simulink model "beluga_control_a"  (R2016a)
settings: Solver=FixedStepAuto  SolverMode=SingleTasking  StartTime=0.0  StopTime=10.0  FixedStep=0.001  RelTol=1e-3
values from neighbouring files (symbols this model uses):
  Ix = 0.05    [belugaSimulation.m]    (also in belugaStep.m; iverSimulation.m = 0; matlab.mat)
  Iy = 2.05    [belugaSimulation.m]    (also in belugaStep.m; iverSimulation.m = 0; matlab.mat)
  Iz = 2.06    [belugaSimulation.m]    (also in belugaStep.m; iverSimulation.m = 0; matlab.mat)
  K_pdot = -0.0704    [belugaSimulation.m]    (also in belugaStep.m; iverSimulation.m = 0; matlab.mat)
  m = 16.7/2.2    (= 7.59090909091)    [belugaSimulation.m]    (also in belugaStep.m = 4.2173; gps_state_est.m = 1; iverSimulation.m = 0; lin_test.m = 20.2)
  M_qdot = -3.2455    [belugaSimulation.m]    (also in belugaStep.m; iverSimulation.m = 0; matlab.mat)
  M_wdot = 2.5656    [belugaSimulation.m]    (also in belugaStep.m; iverSimulation.m = 0; matlab.mat)
  N_rdot = -3.2455    [belugaSimulation.m]    (also in belugaStep.m; iverSimulation.m = 0; matlab.mat)
  N_vdot = -2.5656    [belugaSimulation.m]    (also in belugaStep.m; iverSimulation.m = 0; matlab.mat)
  X_udot = -0.51334    [belugaSimulation.m]    (also in belugaStep.m; iverSimulation.m = 0; matlab.mat)
  xg = 0    [belugaSimulation.m]    (also in belugaStep.m; iverSimulation.m; matlab.mat)
  Y_rdot = -2.5656    [belugaSimulation.m]    (also in belugaStep.m; iverSimulation.m = 0; matlab.mat)
  Y_vdot = -23.8314    [belugaSimulation.m]    (also in belugaStep.m; iverSimulation.m = 0; matlab.mat)
  Z_qdot = 2.5656    [belugaSimulation.m]    (also in belugaStep.m; iverSimulation.m = 0; matlab.mat)
  Z_wdot = -23.8314    [belugaSimulation.m]    (also in belugaStep.m; iverSimulation.m = 0; matlab.mat)
  zg = 0    [belugaSimulation.m]    (also in belugaStep.m; iverSimulation.m; matlab.mat)
libraries: dspinverses x1
settings Model: Creator=HMCLoaner  LastModifiedBy=chriskotcherha
settings DebuggingCC: SFUnexpectedBacktrackingDiag=error  SFNoUnconditionalDefaultTransitionDiag=error
settings GRTTargetCC: TargetLangStandard=C99 (ISO)  GeneratePreprocessorConditionals=Use local settings
settings ConfigComp: CovMetricSettings=dwe  CovHtmlReporting=off  CovSaveCumulativeToWorkspaceVar=off  CovSaveSingleToWorkspaceVar=off  CovExternalEMLEnable=on

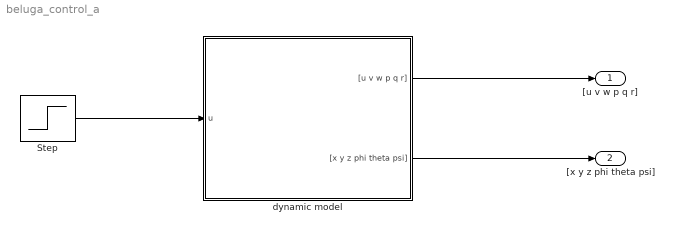
== system beluga_control_a ==
  Step : Step  Time=0  Before=[0 0 0 0]  After=1*[1 1 1 1]  SampleTime=0
  "dynamic model " : Subsystem
  "[u v w p q r]" : Outport
  "[x y z phi theta psi]" : Outport  Port=2
  wires:
  Step/1 -> "dynamic model "/1(u)
  "dynamic model "/1("[u v w p q r]") -> "[u v w p q r]"/1
  "dynamic model "/2("[x y z phi theta psi]") -> "[x y z phi theta psi]"/1

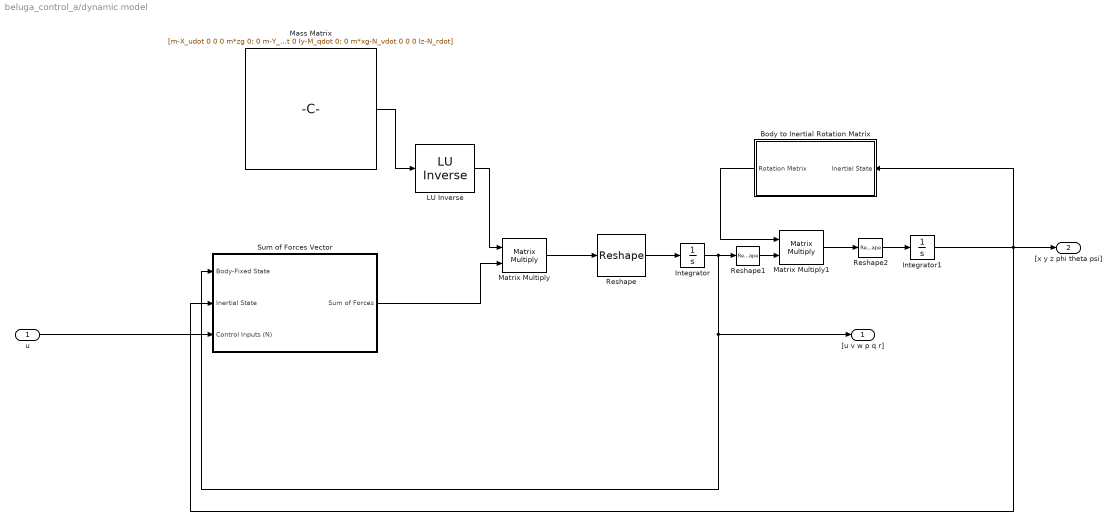
== system beluga_control_a/dynamic model  ==
  u : Inport  PortDimensions=[4,1]
  " LU Inverse" : dspinverses/ LU Inverse
  Body to Inertial Rotation Matrix : Subsystem
  Integrator : Integrator  InitialCondition=[0 0 0 0 0 0]'
  Integrator1 : Integrator  InitialCondition=[0 0 0 0 0 0]'
  "Mass Matrix " : Constant  Value=[m-X_udot 0 0 0 m*zg 0; 0 m-Y_vdot 0 -m*zg 0 m*xg-Y_rdot; 0 0 m-Z_wdot 0 -m*xg-Z_qdot 0; 0 -m*zg 0 Ix-K_pdot 0 0; m*zg 0 -m*xg-M_wdot 0 Iy-M_qdot 0; 0 m*xg-N_vdot 0 0 0 Iz-N_rdot]  VectorParams1D=off
  Matrix Multiply : Product  Multiplication=Matrix(*)
  Matrix Multiply1 : Product  Multiplication=Matrix(*)
  Reshape : Reshape  OutputDimensions=3
  Reshape1 : Reshape  OutputDimensions=[1,6]
  Reshape2 : Reshape  OutputDimensions=[6,1]
  Sum of Forces Vector : Subsystem
  "[u v w p q r]" : Outport
  "[x y z phi theta psi]" : Outport  Port=2
  wires:
  Matrix Multiply/1 -> Reshape/1
  Integrator/1 -> "[u v w p q r]"/1, Sum of Forces Vector/1(Body-Fixed State), Reshape1/1
  " LU Inverse"/1 -> Matrix Multiply/1
  Reshape1/1 -> Matrix Multiply1/2
  Matrix Multiply1/1 -> Reshape2/1
  Reshape2/1 -> Integrator1/1
  "Mass Matrix "/1 -> " LU Inverse"/1
  Body to Inertial Rotation Matrix/1(Rotation Matrix) -> Matrix Multiply1/1
  Sum of Forces Vector/1(Sum of Forces) -> Matrix Multiply/2
  u/1 -> Sum of Forces Vector/3(Control Inputs (N))
  Integrator1/1 -> "[x y z phi theta psi]"/1, Sum of Forces Vector/2(Inertial State), Body to Inertial Rotation Matrix/1(Inertial State)
  Reshape/1 -> Integrator/1

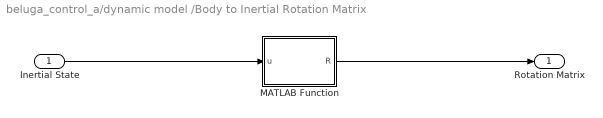
== system beluga_control_a/dynamic model /Body to Inertial Rotation Matrix ==
  Inertial State : Inport
  MATLAB Function : MATLAB Function  TreatAsAtomicUnit=on
  Rotation Matrix : Outport  PortDimensions=[6,6]
  wires:
  MATLAB Function/1(R) -> Rotation Matrix/1
  Inertial State/1 -> MATLAB Function/1(u)

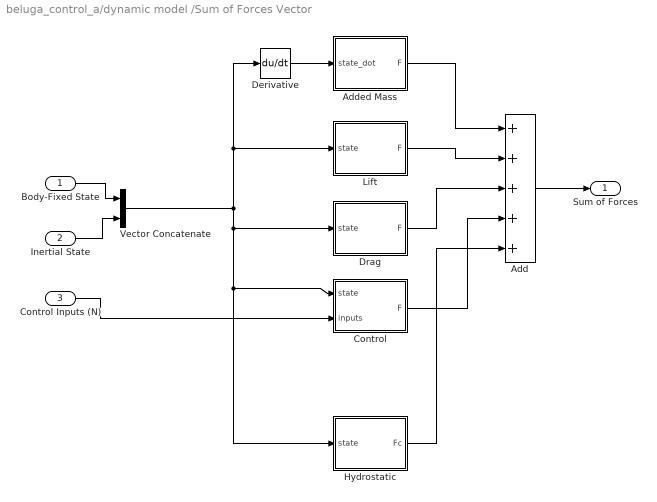
== system beluga_control_a/dynamic model /Sum of Forces Vector ==
  Body-Fixed State : Inport
  Inertial State : Inport  Port=2
  Control Inputs (N) : Inport  Port=3
  Add : Sum  Inputs=+++++
  Added Mass : MATLAB Function  TreatAsAtomicUnit=on
  Control : MATLAB Function  TreatAsAtomicUnit=on
  Derivative : Derivative
  Drag : MATLAB Function  TreatAsAtomicUnit=on
  Hydrostatic : MATLAB Function  TreatAsAtomicUnit=on
  Lift : MATLAB Function  TreatAsAtomicUnit=on
  Vector Concatenate : Concatenate
  Sum of Forces : Outport
  wires:
  Body-Fixed State/1 -> Vector Concatenate/1
  Inertial State/1 -> Vector Concatenate/2
  Vector Concatenate/1 -> Drag/1(state), Control/1(state), Hydrostatic/1(state), Derivative/1, Lift/1(state)
  Control Inputs (N)/1 -> Control/2(inputs)
  Hydrostatic/1(Fc) -> Add/5
  Add/1 -> Sum of Forces/1
  Control/1(F) -> Add/4
  Drag/1(F) -> Add/3
  Lift/1(F) -> Add/2
  Added Mass/1(F) -> Add/1
  Derivative/1 -> Added Mass/1(state_dot)

== matlab function beluga_control_a/dynamic model /Sum of Forces Vector/Control ==
  data: state input; F output; inputs input
function F = fcn(state, inputs)
    
    %% Constants TODO
        % TODO #1: Add in multiplying the sum of forces by r when
        %           calculating K_c
        % TODO #2: Check constants and polarity for K_c
        % TODO #3: Check M_c
        % TODO #4: Check polarity of N_c
        % TODO #5: Add in multiplying the sum of forces by L when
        %           calculating M_c
        % TODO #6: Add in multiplying the sum of forces by L when
        %           calculating N_c    
    %% Thruster Model
    % Values from documentation stationary calibration
    thruster_pwm = [1100        1110        1120        1130        1140        1150        1160        1170 1180        1190        1200        1210        1220        1230        1240        1250        1260        1270        1280        1290        1300        1310        1320        1330        1340        1350        1360        1370        1380        1390        1400        1410         1420        1430        1440        1450        1460        1470        1480        1490 1500        1510        1520        1530        1540        1550        1560        1570 1580        1590        1600        1610        1620        1630        1640        1650 1660        1670        1680        1690        1700        1710        1720        1730 1740        1750        1760        1770        1780        1790        1800        1810 1820        1830        1840        1850        1860        1870        1880        1890 1900];
    thruster_force = 9.81*[-4.0823   -4.0823   -4.0869   -3.8283   -3.7331   -3.6197   -3.4428   -3.3022   -3.1842   -3.0572 -2.9075   -2.8168   -2.7079   -2.5265   -2.3632   -2.2589   -2.1772   -1.9913   -1.8824   -1.7690 -1.6420   -1.4923   -1.3336   -1.2428   -1.1204   -1.0251   -0.9072   -0.7893   -0.6940   -0.6169 -0.5216   -0.4354   -0.3538   -0.2767   -0.1905   -0.1134   -0.0544   -0.0272         0         0 0         0         0    0.0590    0.1134    0.1860    0.2631    0.3493    0.4173    0.5216 0.6350    0.7167    0.8437    0.9435    1.1022    1.2474    1.3925    1.5286    1.6783    1.8053 1.9595    2.0956    2.2181    2.4131    2.5220    2.6943    2.8259    3.0209    3.1933    3.3521 3.4473    3.4927    3.7784    3.9417    4.0052    4.1957    4.3772    4.5677    4.8035    4.8988 5.0938];
    
    
    % From Arduino implementation
    DEAD_POS = 16;
    DEAD_NEG = -35;
    PERIOD = 500; % [ms]
    LEAK_THRESH = 150;
    
    %Correct for deadzone
    for i = 1:numel(inputs)
        if inputs(i) > 0
            inputs(i) = inputs(i)*50+DEAD_POS;
        elseif inputs(i) < 0
            inputs(i) = inputs(i)*50+DEAD_NEG;            
        end
        
        inputs(i) = inputs(i) + 1500;
        inputs(i) = interp1(thruster_pwm, thruster_force, inputs(i)); % assuming static thrust
    end


    %% States and calculations
    % defining states
    u = state(1); % x - velocity
    v = state(2); % y - velocity
    w = state(3); % z - velocity
    p = state(4); % angular velocity around the x-axis (velocity of phi)
    q = state(5); % angular velocity around the y-axis (velocity of theta)
    r = state(6); % angular velocity around the z-axis (velocity of psi)
    
    x = state(7); % x - position
    y = state(8); % y - position
    z = state(9); % z - position
    phi = state(10);   % rotation of the y-axis in the inertial frame
    theta = state(11); % rotation of the z-axis in the inertial frame
    psi = state(12);   % rotation of the x-axis in the inertial axis
    
    %approximate dynamic thrust
    d = 0.076; % diameter of the propeller (in meters)
    rho = 1000; % fluid density of water (in kg/m^3)
    for i = 1:numel(inputs)
        if inputs(i)==0
            inputs(i) = 0.0001;
        end
        n = sqrt(abs(inputs(i))/(rho*d^4*0.1858));
            %   n is the desired propeller speed, from the equation for thrust,
            %   abs(inputs(i)) is the thrust, and 0.1858 is the propeller
            %   constant for static thrust, derived from Blue Robotics data
            %   
            %   This gives static thrust, but can be used as K value to
            %   calculate dynamic thrust and dynamic value for propeller
            %   constant
        Kt = 0.1858*(1-(u/(n*d))); 
            %   Now the dynamic propeller constant can be calculated,
            %   where u is the x - velocity of the AUV  
        Kt(isnan(Kt))=0; % if the dynamic propeller constant is a NaN, it is reset
                         % to zero
        inputs(i) = real(Kt*rho*n.^2*d^4);  % Now store in the array the real portion
                                            % of the dynamic value for the
                                            % required thrust
    end
    
    % Control Forces
    X_c = sum(inputs); % Forward thrust (along the x-axis of the AUV
                       % is the sum of the thrust from each propeller
    Y_c = 0; % There is no thrust along the y-axis of the AUV
    Z_c = 0; % There is no thrust along the z-axis of the AUV
    K_c = inputs(1)-inputs(2)+inputs(3)-inputs(4); 
        % The moment about the x-axis of the AUV is sum of the thrusts from
        % thrusters 1 and 3 minus the sum of the thrust from thrusters 2
        % and 4
    M_c = inputs(2)-inputs(4); % 
        % The moment about the y-axis of the AUV is the thrust from the 
        % first thruster minus the thrust from the third thruster
    N_c = inputs(1)-inputs(3); 
        % The moment about the z-axis of the AUV is the thrust from the 
        % second thruster minus the thrust from the fourth thruster 
    
    % output force vector
    X = X_c;    % The new force for the X-axis
    Y = Y_c;    % The new force for the Y-axis
    Z = Z_c;    % The new force for the Z-axis
    K = K_c;    % The new moment for the X-axis
    M = M_c;    % The new moment for the y-axis
    N = N_c;    % The new moment for the Z-axis
    F = [X Y Z K M N]'; % The output control forces and moments
    % For Troubleshooting Purposes: 
    %F = [0 0 0 0 0 0]';
end

== matlab function beluga_control_a/dynamic model /Body to Inertial Rotation Matrix/MATLAB Function ==
  data: u input; R output
function R = fcn(u)
    % Inputs
    x = u(1);
    y = u(2);
    z = u(3);
    phi = u(4);
    theta = u(5);
    psi = u(6);
    
    % transformation
    cosphi = cos(phi);
    sinphi = sin(phi);
    costheta = cos(theta);
    sintheta = sin(theta);
    cospsi = cos(psi);
    sinpsi = sin(psi);

    R = zeros(6,6);
    R(1,1) = cospsi.*cosphi-costheta.*sinphi.*sinpsi;
    R(1,2) = sinphi.*cospsi+costheta.*cosphi.*sinpsi;
    R(1,3) = sintheta.*sinpsi;

    R(2,1) = -cosphi.*sinpsi-costheta.*cospsi.*sinphi;
    R(2,2) = -sinpsi.*sinphi+costheta.*cosphi.*cospsi;
    R(2,3) = sintheta.*cospsi;

    R(3,1) = sinphi.*sintheta;
    R(3,2) = -cosphi.*sintheta;
    R(3,3) = costheta;
    
    R(4,4) = 1;
    R(5,5) = 1;
    R(6,6) = 1;
end

== matlab function beluga_control_a/dynamic model /Sum of Forces Vector/Hydrostatic ==
  data: state input; Fc output
function Fc = fcn(state)
    %% Constants
    %Measured Parameters:
    W = 198; %N, Weight Force of AUV w/ Ballast
    B = W; %N, Buoyant Force of AUV w/ Ballast
    
    %Measured or Estimated Centers of Buoyancy and Gravity
    zcg = -0.03; %cg right under cb
    
    %% States and calculations
    % defining relevant states
    phi = state(10);
    theta = state(11);
    
    % Hydrostatic forces
    X_hs = -(W-B)*sin(theta); %equation 21, ~0
    Y_hs = (W-B)*cos(theta)*sin(phi); %equation 21, ~0
    Z_hs = (W-B)*cos(theta)*cos(phi); %equation 21, ~0
    K_hs = -zcg*W*cos(theta)*sin(phi); %equation 24
    M_hs = -zcg*W*sin(theta); %equation 25
    N_hs = 0; %equation 26
    
    % output force vector
    X = X_hs;
    Y = Y_hs;
    Z = Z_hs;
    K = K_hs;
    M = M_hs;
    N = N_hs;
    Fc = [X Y Z K M N]'; 
end

== matlab function beluga_control_a/dynamic model /Sum of Forces Vector/Drag ==
  data: state input; F output
function F = fcn(state)
    %% States and calculations
    % defining states
    u = state(1);
    v = state(2);
    w = state(3);

    q = state(5);
    r = state(6);

    %Drag Constants (pre-calculated, mid-year paper)
    X_u_abs_u = -1.05; %kg*m, Axial
    M_w_abs_w = -74.7; %kg*m/rad^2, Pitch-Z
    M_q_abs_q = -70.3; %kg*m^2/rad^2, Pitch-Pitch
    N_v_abs_v = 74.7; %kg*m/rad^2, Yaw-Y
    N_r_abs_r = -70.3; %kg*m^2/rad^2, Yaw-Yaw
    
    % Drag forces
    X_drag = X_u_abs_u*u*abs(u);
    M_drag = M_w_abs_w*w*abs(w)+M_q_abs_q*q*(abs(q));
    N_drag = N_v_abs_v*v*abs(v)+N_r_abs_r*r*abs(r);
    

    % output force vector
    X = X_drag;
    Y = 0; %negligible
    Z = 0; %negligible
    K = 0; %negligible
    M = M_drag;
    N = N_drag;
    F = [X Y Z K M N]'; 
end

== matlab function beluga_control_a/dynamic model /Sum of Forces Vector/Lift ==
  data: state input; F output
function F = fcn(state)
    
    %% Constants
    %disp('Calc Nonlinear Coeffs')
    %Conversion Factors:
    i2m = 0.0254; %Conversion factor (inches to meters)
    lb2N = 4.44822162; %Conversion factor (lbs-force to Newtons)
    %Water Characteristics:
    %U = 1.5; %nominal velocity (m/s)
    U = 1; %2 knots
    rho = 1.03*10^(3); %seawater density (kg/m^3)
    %****Iver2 Hull Parameters*********************
    a = 8*i2m;
    a_offset = 0*i2m;
    b = 33.375*i2m;
    c = 7.34*i2m;
    c_offset = 1.04*i2m;
    d = 5.83*i2m;
    l = 47.67*i2m;
    Tail_angle = 35.5*pi/180;
    n = 2;
    %****************************************
    %**********Iver2 Moments of Inertia *****
    I_x = 0.05; %kg*m^2
    Iyy = 2.05; %kg*m^2
    Izz = 2.06; %kg*m^2
    %***************************************
    %Measured Parameters:
    W = 41.33*lb2N;
    m = W/9.8;
    B = 41.77*lb2N;
    %Measured or Estimated Centers of Buoyancy and Gravity
    xcg = 0*i2m;
    ycg = 0*i2m;
    zcg = 0.089*i2m;
    xcb = -23.72*i2m;
    ycb = 0*i2m;
    zcb = 0.03*i2m;
    %Vehicle parameters wrt. origin at the center of buoyancy
    x_g = 0;
    y_g = 0;
    z_g = 10*(zcg - zcb); %better COG-COB separation
    x_b = 0;
    y_b = 0;
    z_b = 0;

    %***********************Calculate The Non-Linear Coefficients**************
    %**************************************************************************
    %*****************************Axial Drag***********************************
    %Theoretical Drag Coeffecient: ( REMUS Eq 4.7)
    css = 3.397*10^(-3); %Schoenherr's value for flat plate skin friction
    Ap = l*d; %vehicle plan area
    Af = pi*(d/2)^2; %vehicle frontal area
    Cd = css*pi*Ap/Af*(1+60*(d/l)^3+0.0025*(l/d)); %drag coefficient estimate
    X_u_abs_u = -1/2*rho*Cd*Af; %Linear axial drag coefficient (kg/s)
    %*****************************Crossflow Drag*******************************
    %Define integration step size and limits of integration
    dx = 0.01; %integration step size
    %****Iver2 Values*****
    xn = abs(xcb)-(a-a_offset);
    xn2 = xn + (a-a_offset);
    xt2 = -(b-xn);
    xt = xt2 - (c - c_offset);
    xf = xt;
    xf2 = xt;
    lf = a+b-a_offset; %vehicle forward length
    %*********************
    Cdc = 1.1; %crossflow drag coefficient of a cylinder(Hoerner)
    Cdf = 0.1; %control fin crossflow drag coefficient
    intg = cdrag(xt,xt2,xn,xn2,d,a,a_offset,n,c,Tail_angle,l,lf,dx,xcb);
    Z_w_abs_w = -1/2*rho*Cdc*intg;
    Y_v_abs_v = Z_w_abs_w;
    intg = cdrag(xt,xt2,xn,xn2,d,a,a_offset,n,c,Tail_angle,l,lf,dx,xcb);
    M_w_abs_w = -1/2*rho*Cdc*intg;
    N_v_abs_v = -M_w_abs_w;
    intg = cdrag(xt,xt2,xn,xn2,d,a,a_offset,n,c,Tail_angle,l,lf,dx,xcb);
    Zq_abs_q = 1/2*rho*Cdc*intg;
    intg = cdrag(xt,xt2,xn,xn2,d,a,a_offset,n,c,Tail_angle,l,lf,dx,xcb);
    %*****************************Added Mass***********************************
    %Define axial added mass parameters:
    alpha = 0.03585; %From table 4.1 of REMUS
    %Calculate coefficients
    Xu_dot = -4*alpha*rho*pi/3*(l/2)*(d/2)^2;
    %intg = cdrag(xt,xf,xf2,xt2,xn,xn2,d,a,a_offset,n,c,l,lf,rho,afin,...
     %dx,Tail_angle,xcb);
    Yv_dot = intg;
    Zw_dot = Yv_dot;
    %intg = cdrag(xt,xf,xf2,xt2,xn,xn2,d,a,a_offset,n,c,l,lf,rho,afin,...
     %dx,Tail_angle,xcb);
    Mw_dot = intg; %Actual Equations in 4.20
    Nv_dot = -Mw_dot;
    Yr_dot = Nv_dot;
    Zq_dot = Mw_dot;
    %intg = cdrag(xt,xf,xf2,xt2,xn,xn2,d,a,a_offset,n,c,l,lf,rho,afin,...
     %dx,Tail_angle,xcb);
    Mq_dot = intg;
    Nr_dot = Mq_dot;
    %Rolling added mass:
    Kp_dot = -7.04*10^(-2); %kg*m^2/rad
    %Added mass cross-terms:
    X_wq = Zw_dot; %kg/rad
    X_qq = Zq_dot; %kg*m/rad
    X_vr = -Yv_dot; %kg/rad;
    X_rr = -Yr_dot; %kg*m/rad
    Yura = Xu_dot; %kg/rad
    Y_wp = -Zw_dot; %kg/rad
    Y_pq = -Zq_dot; %kg*m/rad
    Zuqa = -Xu_dot; %kg/rad
    Z_vp = Yv_dot; %kg/rad
    Z_rp = Yr_dot; %kg/rad
    Muwa = -(Zw_dot - Xu_dot); %kg
    M_vp = -Yr_dot; %kg*m/rad
    M_rp = (Kp_dot - Nr_dot); %kg*m^2/rad^2
    Muqa = -Zq_dot; %kg*m/rad
    Nuva = -(Xu_dot - Yv_dot); %kg
    N_wp = Zq_dot; %kg*m/rad
    N_pq = -(Kp_dot - Mq_dot); %kg*m^2/rad^2
    Nura = Yr_dot; %kg*m/rad
    %***************************Body Lift Force/Moment*************************
    cydb = (l/d)*0.003*180/pi;
    xcp = -0.65*l - xcb;
    Zuwl = -1/2*rho*d^2*cydb;
    Muwl = -1/2*rho*d^2*cydb*xcp;
    Yuvl = -1/2*rho*d^2*cydb;
    Nuvl = 1/2*rho*d^2*cydb*xcp;
    

    %*********************Combine Like Terms**********************************
    %The following equations combine the like terms as shown in Section 4.7 of
    %the Remus paper.
    Y_uv = Yuvl;
    Y_ur = Yura;
    Z_uw = Zuwl;
    Z_uq = Zuqa;
    M_uw = Muwa + Muwl;
    M_uq = Muqa;
    N_uv = Nuva + Nuvl;
    N_ur = Nura;

    
    %% States and calculations
    % defining states
    u = state(1);
    v = state(2);
    w = state(3);
    p = state(4);
    q = state(5);
    r = state(6);

       
    % Lift forces
    X_lift = X_wq*w*q+X_qq*q^2+X_vr*v*r+X_rr*r^2;
    Y_lift = Y_wp*w*p+Y_pq*q*p+Y_ur*u*r+Y_uv*u*v;
    Z_lift = Z_uq*u*q+Z_vp*v*p+Z_rp*r*p+Z_uw*u*w;
    K_lift = 0;
    M_lift = M_uq*u*q+M_vp*v*p+M_rp*r*p+M_uw*u*w;
    N_lift = N_ur*u*r+N_wp*w*p+N_pq*p*q+N_uv*u*v;
    

    % output force vector
    X = X_lift;
    Y = Y_lift;
    Z = Z_lift;
    K = K_lift;
    M = M_lift;
    N = N_lift;
    F = [X Y Z K M N]'; 
    F = [0 0 0 0 0 0]';
end

function intg = cdrag(xt,xt2,xn,xn2,d,a,a_offset,n,c,theta,l,lf,dx,xb)
%This function performs the integration for the first equation of 4.8 in
%the REMUS thesis
intg = 0;
xti = l;
for x = xt:dx:xt2
 %Need to adjust for the difference in origin definitions between the
 %radius functions and the body-coord with the following transform:
 Rx = ( 1/2*d - ( 3*d/(2*c^2) - tan(theta)/c )*(xti-lf)^2 + ...
 ( d/(c^3) - tan(theta)/(c^2) )*(xti - lf)^3 );
 xti = xti-dx;

 intg = intg + 2*Rx*dx;
end
for x = xt2:dx:xn
 Rx = d/2;
 intg = intg + 2*Rx*dx;
end
for x = xn:dx:xn2
 %Need to adjust for the difference in origin definitions betwee the
 %radius functions and the body-coord with the following transform:
 xi = -( x - abs(xb) + (a-a_offset) ) + a;
 Rx = ( 1/2*d*( 1 - ( (xi + a_offset-a)/a )^2 )^(1/n) );

 intg = intg + 2*Rx*dx;
end
end
%End of cdrag function

== matlab function beluga_control_a/dynamic model /Sum of Forces Vector/Added Mass ==
  data: state_dot input; F output
function F = fcn(state_dot)
    
    %% Constants
    %disp('Calc Nonlinear Coeffs')
    %Conversion Factors:
    i2m = 0.0254; %Conversion factor (inches to meters)
    lb2N = 4.44822162; %Conversion factor (lbs-force to Newtons)
    %Water Characteristics:
    %U = 1.5; %nominal velocity (m/s)
    U = 1; %2 knots
    rho = 1.03*10^(3); %seawater density (kg/m^3)
    %****Iver2 Hull Parameters*********************
    a = 0.152;
    a_offset = 0.000001;
    b = 1.088;
    c = 0.00001;
    c_offset = 0;
    d = 0.1397;
    l = a+b+c;
    Tail_angle = 0.1;
    n = 0.1;
    %****************************************
    %**********Iver2 Moments of Inertia *****
    I_x = 0.05; %kg*m^2
    Iyy = 2.05; %kg*m^2
    Izz = 2.06; %kg*m^2
    %***************************************
    %Measured Parameters:
    W = 41.33*lb2N;
    m = W/9.8;
    B = 41.77*lb2N;
    %Measured or Estimated Centers of Buoyancy and Gravity
    xcg = 0*i2m;
    ycg = 0*i2m;
    zcg = 0.089*i2m;
    xcb = -23.72*i2m;
    ycb = 0*i2m;
    zcb = 0.03*i2m;
    %Vehicle parameters wrt. origin at the center of buoyancy
    x_g = 0;
    y_g = 0;
    z_g = 10*(zcg - zcb); %better COG-COB separation
    x_b = 0;
    y_b = 0;
    z_b = 0;
    %Fin characteristic parameters:
    fin1 = 2.54*i2m;
    fin2 = 1.92*i2m;
    fin3 = 5.7*i2m;
    fin4 = 1.26*i2m;
    fin5 = 3.51*i2m;
    fin6 = 4.5*i2m;
    %***********************Calculate The Non-Linear Coefficients**************
    %**************************************************************************
    %*****************************Axial Drag***********************************
    %Theoretical Drag Coeffecient: ( REMUS Eq 4.7)
    css = 3.397*10^(-3); %Schoenherr's value for flat plate skin friction
    Ap = l*d; %vehicle plan area
    Af = pi*(d/2)^2+4*pi*(0.05)^2; %vehicle frontal area
    Cd = css*pi*Ap/Af*(1+60*(d/l)^3+0.0025*(l/d)); %drag coefficient estimate
    X_u_abs_u = -1/2*rho*Cd*Af; %Linear axial drag coefficient (kg/s)
    %*****************************Crossflow Drag*******************************
    %Define integration step size and limits of integration
    dx = 0.01; %integration step size
    %****Iver2 Values*****
    xn = abs(xcb)-(a-a_offset);
    xn2 = xn + (a-a_offset);
    xt2 = -(b-xn);
    xt = xt2 - (c - c_offset);
    xf = xt + fin4;
    xf2 = xt+fin6;
    lf = a+b-a_offset; %vehicle forward length
    %*********************
    Cdc = 1.1; %crossflow drag coefficient of a cylinder(Hoerner)
    taper = (fin5 - fin4)/(fin6 - fin4); %fin taper ratio
    Cdf = 0.1 + 0.7*taper; %control fin crossflow drag coefficient
    Sfin = 1/2*(fin1-fin2)*(fin6-fin4)+1/2*(fin6-fin5)*(fin3-fin1)+...
     (fin6-fin4)*(fin3-fin1); %control fin planform area
    xfin = xf2; %fin moment arm wrt origin at COB
    intg = cdrag(xt,xt2,xn,xn2,d,a,a_offset,n,c,Tail_angle,l,lf,dx,xcb);
    Z_w_abs_w = -1/2*rho*Cdc*intg - 2*(1/2*rho*Sfin*Cdf);
    Y_v_abs_v = Z_w_abs_w;
    intg = cdrag(xt,xt2,xn,xn2,d,a,a_offset,n,c,Tail_angle,l,lf,dx,xcb);
    M_w_abs_w = -1/2*rho*Cdc*intg - 2*xfin*(1/2*rho*Sfin*Cdf);
    N_v_abs_v = -M_w_abs_w;
    intg = cdrag(xt,xt2,xn,xn2,d,a,a_offset,n,c,Tail_angle,l,lf,dx,xcb);
    Zq_abs_q = 1/2*rho*Cdc*intg + 2*xfin*abs(xfin)*(1/2*rho*Sfin*Cdf);
    Y_r_abs_r = -Zq_abs_q;
    intg = cdrag(xt,xt2,xn,xn2,d,a,a_offset,n,c,Tail_angle,l,lf,dx,xcb);
    M_q_abs_q = -1/2*rho*Cdc*intg - 2*(xfin^3)*(1/2*rho*Sfin*Cdf);
    N_r_abs_r = M_q_abs_q;
    %Rolling Drag
    K_p_abs_p = -1.3*10^(-1); %Used REMUS VALUE
    %*****************************Added Mass***********************************
    %Define axial added mass parameters:
    alpha = 0.5*(0.03585+0.02071); %From table 4.1 of REMUS
    afin = fin3; %max fin height above the centerline
    %Calculate coefficients
    rho = 1000;
    l = 1.24;
    d = 0.14;
    alpha = 0.0265;
    
    Xu_dot = -4*alpha*rho*pi/3*(l/2)*(d/2)^2;
    %intg = cdrag(xt,xf,xf2,xt2,xn,xn2,d,a,a_offset,n,c,l,lf,rho,afin,...
     %dx,Tail_angle,xcb);
    Yv_dot = intg;
    Zw_dot = Yv_dot;
    %intg = cdrag(xt,xf,xf2,xt2,xn,xn2,d,a,a_offset,n,c,l,lf,rho,afin,...
     %dx,Tail_angle,xcb);
    Mw_dot = intg; %Actual Equations in 4.20
    Nv_dot = -Mw_dot;
    Yr_dot = Nv_dot;
    Zq_dot = Mw_dot;
    %intg = cdrag(xt,xf,xf2,xt2,xn,xn2,d,a,a_offset,n,c,l,lf,rho,afin,...
     %dx,Tail_angle,xcb);
    Mq_dot = intg;
    Nr_dot = Mq_dot;
    %Rolling added mass:
    Kp_dot = -7.04*10^(-2); %kg*m^2/rad
    %Added mass cross-terms:
    X_wq = Zw_dot; %kg/rad
    X_qq = Zq_dot; %kg*m/rad
    X_vr = -Yv_dot; %kg/rad;
    X_rr = -Yr_dot; %kg*m/rad
    Yura = Xu_dot; %kg/rad
    Y_wp = -Zw_dot; %kg/rad
    Y_pq = -Zq_dot; %kg*m/rad
    Zuqa = -Xu_dot; %kg/rad
    Z_vp = Yv_dot; %kg/rad
    Z_rp = Yr_dot; %kg/rad
    Muwa = -(Zw_dot - Xu_dot); %kg
    M_vp = -Yr_dot; %kg*m/rad
    M_rp = (Kp_dot - Nr_dot); %kg*m^2/rad^2
    Muqa = -Zq_dot; %kg*m/rad
    Nuva = -(Xu_dot - Yv_dot); %kg
    N_wp = Zq_dot; %kg*m/rad
    N_pq = -(Kp_dot - Mq_dot); %kg*m^2/rad^2
    Nura = Yr_dot; %kg*m/rad
    %***************************Body Lift Force/Moment*************************
    cydb = (l/d)*0.003*180/pi;
    xcp = -0.65*l - xcb;
    Zuwl = -1/2*rho*d^2*cydb;
    Muwl = -1/2*rho*d^2*cydb*xcp;
    Yuvl = -1/2*rho*d^2*cydb;
    Nuvl = 1/2*rho*d^2*cydb*xcp;
    %**************************Fin Lift Force**********************************
    %Define Fin Lift coefficients
    SpanAve = 1/2*( (fin3-fin2)+(fin3-fin1) ); %avg span of one fin
    ARe = 2*(SpanAve^2)/Sfin; %Effective wing aspect ratio
    Cla = inv( 1/(2*0.9*pi) + 1/(pi*ARe) );
    Yuvf = -1/2*rho*Cla*Sfin; %kg/m
    Y_uudr = -Yuvf; %kg/(m*rad)
    Zuwf = -1/2*rho*Cla*Sfin; %kg/m
    Z_uuds = Zuwf; %kg/(m*rad)
    Zuqf = 1/2*rho*Cla*Sfin*xfin; %kg/rad
    Yurf = -Zuqf; %kg/rad
    Muwf = 1/2*rho*Cla*Sfin*xfin; %kg
    M_uuds = Muwf; %kg/rad
    Nuvf = -1/2*rho*Cla*Sfin*xfin; %kg
    N_uudr = -Nuvf; %kg/rad
    Nurf = -1/2*rho*Cla*Sfin*xfin^2;%kg*m/rad
    Muqf = Nurf; %kg*m/rad
    
    %% States and calculations
    % defining states
    u_dot = state_dot(1);
    v_dot = state_dot(2);
    w_dot = state_dot(3);
    p_dot = state_dot(4);
    q_dot = state_dot(5);
    r_dot = state_dot(6);
    
    x_dot = state_dot(7);
    y_dot = state_dot(8);
    z_dot = state_dot(9);
    phi_dot = state_dot(10);
    theta_dot = state_dot(11);
    psi_dot = state_dot(12);
    
    % Added mass
    X_am = Xu_dot*u_dot;
    Y_am = Yv_dot*v_dot;
    Z_am = Zw_dot*w_dot+Zq_dot*q_dot;
    K_am = Kp_dot*p_dot;
    M_am = Mw_dot*w_dot+Mq_dot*q_dot;
    N_am = Nv_dot*v_dot+Nr_dot*r_dot;
    
    % output force vector
    X = X_am;
    Y = Y_am;
    Z = Z_am;
    K = K_am;
    M = M_am;
    N = N_am;
    %F = [X Y Z K M N]'; 
    F = [X 0 0 0 0 0]';
end

function intg = cdrag(xt,xt2,xn,xn2,d,a,a_offset,n,c,theta,l,lf,dx,xb)
%This function performs the integration for the first equation of 4.8 in
%the REMUS thesis
intg = 0;
xti = l;
for x = xt:dx:xt2
 %Need to adjust for the difference in origin definitions between the
 %radius functions and the body-coord with the following transform:
 Rx = ( 1/2*d - ( 3*d/(2*c^2) - tan(theta)/c )*(xti-lf)^2 + ...
 ( d/(c^3) - tan(theta)/(c^2) )*(xti - lf)^3 );
 xti = xti-dx;

 intg = intg + 2*Rx*dx;
end
for x = xt2:dx:xn
 Rx = d/2;
 intg = intg + 2*Rx*dx;
end
for x = xn:dx:xn2
 %Need to adjust for the difference in origin definitions betwee the
 %radius functions and the body-coord with the following transform:
 xi = -( x - abs(xb) + (a-a_offset) ) + a;
 Rx = ( 1/2*d*( 1 - ( (xi + a_offset-a)/a )^2 )^(1/n) );

 intg = intg + 2*Rx*dx;
end
end
%End of cdrag function
